simulink model "CC_Flight_Simulation"  (R2020a)
settings: Solver=VariableStepAuto  StartTime=0.0  StopTime=55  RelTol=1e-3
values from neighbouring files (symbols this model uses):
  Ar = 0.0126676869774    [barrowaman.mat]
  CD_data = [0.48 0.48 0.47 0.46 0.45 0.44 0.43 0.42 0.42 0.41 0.4 0.4 ... (150 elements, 150x1)]    [barrowaman.mat]
  CD_input = [0.01 0.02 0.03 0.04 0.05 0.06 0.07 0.08 0.09 0.1 0.11 0.12 ... (150 elements, 150x1)]    [barrowaman.mat]
  CnalfaBody = 2.2 * lTubo    [Barrowman_Equations.m]    (also in barrowaman.mat = -4.333362)
  CnAlfaNose = 2 * pi * (r0^2) / Ar    [Barrowman_Equations.m]    (also in barrowaman.mat = 2)
  Cnalfat = Cnalfat * (1 + r0/(span + r0))    [Barrowman_Equations.m]    (also in barrowaman.mat = 7.14285935703)
  CnAlfaTail = 0    [Barrowman_Equations.m]    (also in barrowaman.mat = -1.06144212288)
  Cndomega = (N * (c1 + c2 + c3))/(Ar * (Lr))    [Barrowman_Equations.m]
  Cnfdelta = N * Y / span    [Barrowman_Equations.m]    (also in barrowaman.mat = 4.20666666667)
  delta = 0.00872664625997    [barrowaman.mat]
  F_data = [3391.768 3665.504 3532.913 3357.551 3199.297 3139.417 2412.304 2130.013 2031.639 346.448 81.266 0 ... (14 elements, 14x1)]    [barrowaman.mat]
  F_input = [0.02 0.057 0.148 0.496 0.817 0.936 1.173 1.501 1.717 1.78 1.812 1.832 ... (14 elements, 14x1)]    [barrowaman.mat]
  Lr = 0.127    [barrowaman.mat]
  mdescarregado = 15.576    [barrowaman.mat]
  MDot_data = [-1.96086837808 -2.11912220509 -2.04246793537 -1.9410866497 -1.84959593916 -1.81497776997 -1.39461503025 -1.23141533755 -1.1745427962 -0.200290505674 -0.0469819662232 0 ... (18 elements, 18x1)]    [barrowaman.mat]
  MDot_input = [0.02 0.057 0.148 0.496 0.817 0.936 1.173 1.501 1.717 1.78 1.812 1.832 ... (18 elements, 18x1)]    [barrowaman.mat]
  r = 0    [Barrowman_Equations.m]    (also in barrowaman.mat = 1.45977011494)
  x_cg = -1.278    [barrowaman.mat]
  XB = -(logiva - logiva/2)    [Barrowman_Equations.m]    (also in barrowaman.mat = 0.279145)
  Xtail = 0    [Barrowman_Equations.m]    (also in barrowaman.mat = -2.55613084112)
  XTB = pos_aletas - (sweep / 3) * ( (Cr + 2 * Ct) / (Cr + Ct) ) + (1/6) * (Cr + Ct - Cr * Ct / (Cr + Ct))    [Barrowman_Equations.m]    (also in barrowaman.mat = -2.37866666667)
  Y = rt + (span/3) * yparcial    [Barrowman_Equations.m]    (also in barrowaman.mat = 0.105166666667)
undefined symbols (not defined in the file or in its folder): F, Light, MIL
libraries: sharedutil x8, aerolibasang x3, aerolibwind2 x3, aerolibanim x1, aerolibatmos2 x1, shared6dof x1
settings Model: Creator=bruno  LastModifiedBy=patri
settings OptimizationCC: LifeSpan=inf
settings DebuggingCC: ArithmeticOperatorsInVariantConditions=warning
settings SFSimCC: CustomCodeUndefinedFunction=UseInterfaceOnly
settings CodeAppCC: StateflowObjectComments=on
settings SimscapeCC: SimscapeNormalizeSystem=off

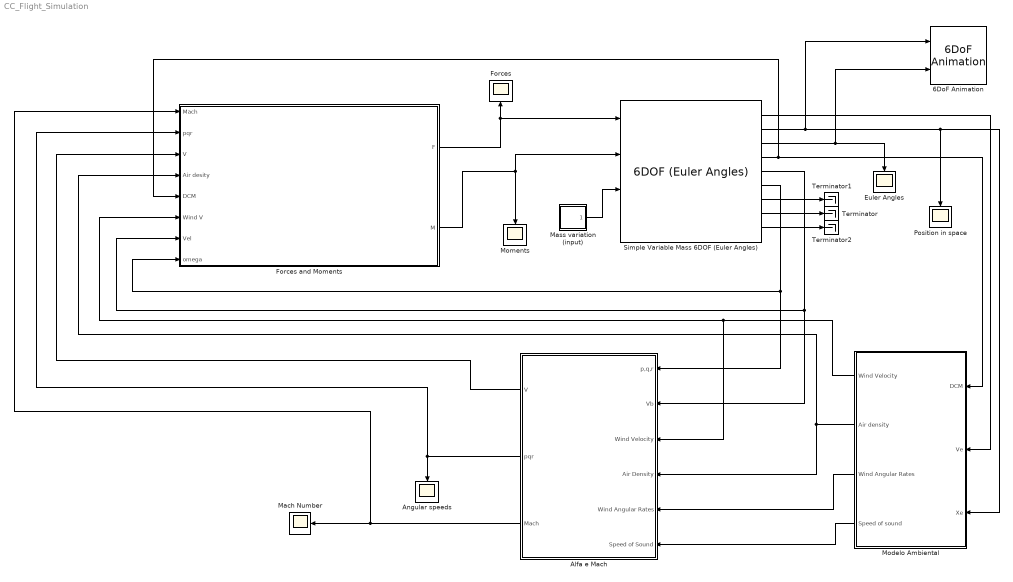
== system CC_Flight_Simulation ==
  6DoF Animation : aerolibanim/6DoF Animation  u1=[0 400 -200 200 0 4000]  u2=0.1  u3=100  u4=[4000 0 -5000]  u5=Fly alongside  u6=[2000 500 -3150]  u7=10  u8=on
  Alfa e Mach : Subsystem
  Angular speeds : Scope
  Euler Angles : Scope
  Forces : Scope
  "Forces and Moments " : Subsystem
  Mach Number : Scope
  Mass variation (input) : Subsystem
  Modelo Ambiental : Subsystem
  Moments : Scope
  "Position in space " : Scope
  Simple Variable Mass 6DOF (Euler Angles) : shared6dof/6DOF (Euler Angles)  units=Metric (MKS)  mtype=Simple Variable  rep=Quaternion  xme_0=[5 0 0]  Vm_0=[20 0 0]  eul_0=[0 -pi/2+pi/30 0]  pm_0=[0 0 0]  mass_0=mcarregado  mass_e=mdescarregado  mass_f=mcarregado  inertia=eye(3)  inertia_e=MatrizDeInerciaDescarregado  inertia_f=MatrizDeInercia  k_quat=1.0  vre_flag=on  abi_flag=off  aMode=aMode  xme_statename=''  Vm_statename=''  eul_statename=''  quat_statename=''  pm_statename=''  mass_statename=''
      settings: SourceProductBaseCode=AE,PW,MT,VE,VP
  Terminator : Terminator
  Terminator1 : Terminator
  Terminator2 : Terminator
  wires:
  Simple Variable Mass 6DOF (Euler Angles)/4 -> Modelo Ambiental/1(DCM), "Forces and Moments "/5(DCM)
  Simple Variable Mass 6DOF (Euler Angles)/1 -> Modelo Ambiental/2(Ve)
  Simple Variable Mass 6DOF (Euler Angles)/2 -> 6DoF Animation/1, "Position in space "/1, Modelo Ambiental/3(Xe)
  Modelo Ambiental/2(Air density) -> Alfa e Mach/4(Air Density), "Forces and Moments "/4(Air desity)
  Modelo Ambiental/1(Wind Velocity) -> Alfa e Mach/3(Wind Velocity), "Forces and Moments "/6("Wind V ")
  Simple Variable Mass 6DOF (Euler Angles)/5 -> "Forces and Moments "/7("Vel "), Alfa e Mach/2(Vb)
  Simple Variable Mass 6DOF (Euler Angles)/6 -> "Forces and Moments "/8(omega), Alfa e Mach/1(p,q,r)
  Modelo Ambiental/4(Speed of sound) -> Alfa e Mach/6(Speed of Sound)
  Modelo Ambiental/3(Wind Angular Rates) -> Alfa e Mach/5(Wind Angular Rates)
  Alfa e Mach/3(Mach) -> "Forces and Moments "/1(Mach), Mach Number/1
  Alfa e Mach/2(pqr) -> "Forces and Moments "/2(pqr), Angular speeds/1
  Alfa e Mach/1(V) -> "Forces and Moments "/3("V ")
  Simple Variable Mass 6DOF (Euler Angles)/3 -> 6DoF Animation/2, Euler Angles/1
  "Forces and Moments "/1(F) -> Simple Variable Mass 6DOF (Euler Angles)/1, Forces/1
  Simple Variable Mass 6DOF (Euler Angles)/7 -> Terminator1/1
  Simple Variable Mass 6DOF (Euler Angles)/8 -> Terminator/1
  Simple Variable Mass 6DOF (Euler Angles)/9 -> Terminator2/1
  "Forces and Moments "/2(M) -> Simple Variable Mass 6DOF (Euler Angles)/2, Moments/1
  Mass variation (input)/1("dM/dt ") -> Simple Variable Mass 6DOF (Euler Angles)/3

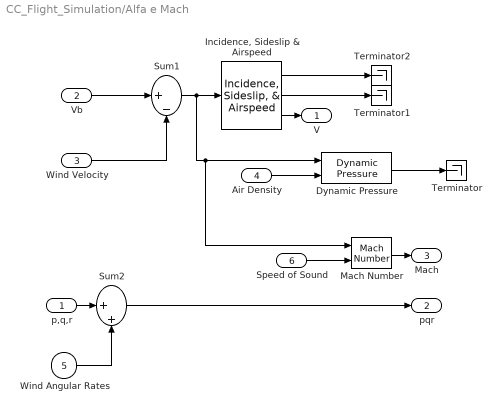
== system CC_Flight_Simulation/Alfa e Mach ==
  p,q,r : Inport
  Vb : Inport  Port=2
  Wind Velocity : Inport  Port=3
  Air Density : Inport  Port=4
  Wind Angular Rates : Inport  Port=5
  Speed of Sound : Inport  Port=6  Unit=m/s
  Dynamic Pressure : aerolibasang/Dynamic Pressure
  "Incidence, Sideslip & Airspeed" : aerolibasang/Incidence, Sideslip, & Airspeed
  Mach Number : aerolibasang/Mach Number
      settings: SourceProductBaseCode=AE
  Sum1 : Sum  Inputs=|+-  InputSameDT=on  SaturateOnIntegerOverflow=on  OutDataTypeStr=Inherit: Same as first input
  Sum2 : Sum  Inputs=|++  InputSameDT=on  SaturateOnIntegerOverflow=on  OutDataTypeStr=Inherit: Same as first input
  Terminator : Terminator
  Terminator1 : Terminator
  Terminator2 : Terminator
  V : Outport  VectorParamsAs1DForOutWhenUnconnected=off
  pqr : Outport  Port=2  VectorParamsAs1DForOutWhenUnconnected=off
  Mach : Outport  Port=3  VectorParamsAs1DForOutWhenUnconnected=off
  wires:
  Wind Velocity/1 -> Sum1/2
  Air Density/1 -> Dynamic Pressure/2
  Dynamic Pressure/1 -> Terminator/1
  "Incidence, Sideslip & Airspeed"/3 -> V/1
  p,q,r/1 -> Sum2/1
  Wind Angular Rates/1 -> Sum2/2
  Sum2/1 -> pqr/1
  Vb/1 -> Sum1/1
  Mach Number/1 -> Mach/1
  Sum1/1 -> Mach Number/1, Dynamic Pressure/1, "Incidence, Sideslip & Airspeed"/1
  Speed of Sound/1 -> Mach Number/2
  "Incidence, Sideslip & Airspeed"/2 -> Terminator1/1
  "Incidence, Sideslip & Airspeed"/1 -> Terminator2/1

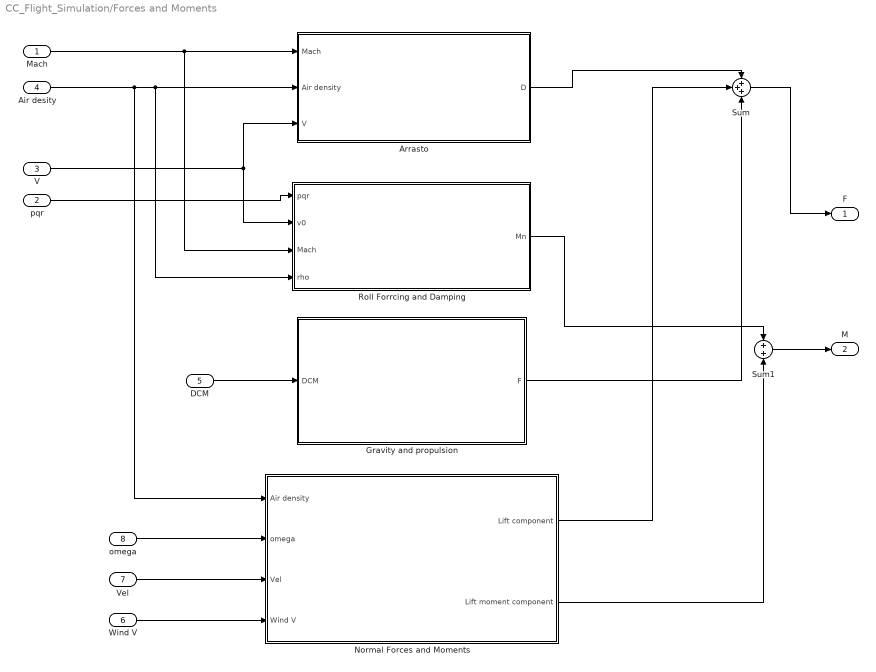
== system CC_Flight_Simulation/Forces and Moments  ==
  Mach : Inport
  pqr : Inport  Port=2
  "V " : Inport  Port=3
  Air desity : Inport  Port=4
  DCM : Inport  Port=5
  "Wind V " : Inport  Port=6
  "Vel " : Inport  Port=7
  omega : Inport  Port=8
  Arrasto : Subsystem
  Gravity and propulsion : Subsystem
  Normal Forces and Moments : Subsystem
  Roll Forrcing and Damping : Subsystem
  Sum : Sum  Inputs=3
  Sum1 : Sum  Inputs=2
  F : Outport  VectorParamsAs1DForOutWhenUnconnected=off
  M : Outport  Port=2  VectorParamsAs1DForOutWhenUnconnected=off
  wires:
  Mach/1 -> Roll Forrcing and Damping/3("Mach "), Arrasto/1(Mach)
  pqr/1 -> Roll Forrcing and Damping/1(pqr)
  "V "/1 -> Roll Forrcing and Damping/2("v0 "), Arrasto/3("V ")
  Air desity/1 -> Roll Forrcing and Damping/4(rho), Arrasto/2(Air density), Normal Forces and Moments/1(Air density)
  Sum/1 -> F/1
  Gravity and propulsion/1(F) -> Sum/3
  DCM/1 -> Gravity and propulsion/1(DCM)
  Arrasto/1(D) -> Sum/1
  Roll Forrcing and Damping/1(Mn) -> Sum1/1
  Sum1/1 -> M/1
  omega/1 -> Normal Forces and Moments/2(omega)
  "Vel "/1 -> Normal Forces and Moments/3("Vel ")
  "Wind V "/1 -> Normal Forces and Moments/4("Wind V ")
  Normal Forces and Moments/1("Lift component ") -> Sum/2
  Normal Forces and Moments/2("Lift moment component ") -> Sum1/2

== system CC_Flight_Simulation/Mass variation (input) ==
  1-D Lookup Table1 : Lookup_n-D  NumberOfTableDimensions=1  BreakpointsForDimension1=MDot_input  Table=MDot_data  InternalRulePriority=Speed  RndMeth=Simplest  InputSameDT=on
  Clock : Clock
  Forças1 : Scope
  "dM/dt " : Outport  VectorParamsAs1DForOutWhenUnconnected=off
  wires:
  1-D Lookup Table1/1 -> "dM/dt "/1, Forças1/1
  Clock/1 -> 1-D Lookup Table1/1

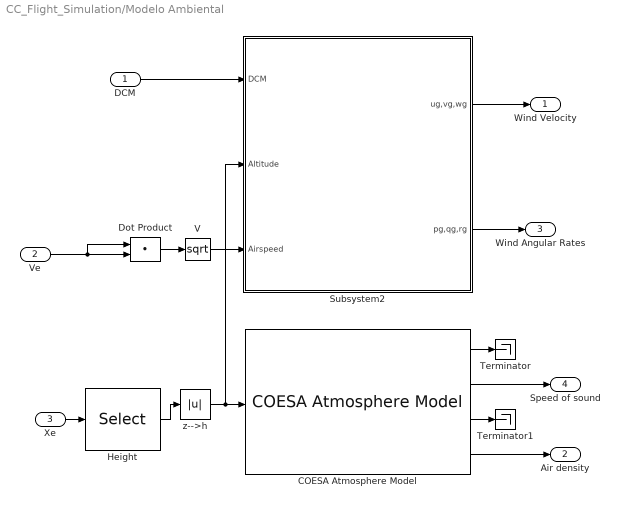
== system CC_Flight_Simulation/Modelo Ambiental ==
  DCM : Inport
  Ve : Inport  Port=2
  Xe : Inport  Port=3
  COESA Atmosphere Model : aerolibatmos2/COESA Atmosphere Model  units=Metric (MKS)  spec=1976 COESA-extended U.S. Standard Atmosphere  model=Profile  profile_var=High temperature  profile_percent=10%  profile_alt=5 km (16404 ft)  envelope_var=High temperature  envelope_percent=1%  action=None
  Dot Product : DotProduct  SaturateOnIntegerOverflow=on  OutDataTypeStr=Inherit: Inherit via internal rule
  Height : Selector  InputPortWidth=3  IndexOptions=Index vector (dialog)  Indices=[3]  OutputSizes=1
  Subsystem2 : Subsystem
  Terminator : Terminator
  Terminator1 : Terminator
  V : Math  Operator=sqrt  SignedPower=on  SaturateOnIntegerOverflow=on
  z-->h : Abs  SaturateOnIntegerOverflow=on
  Wind Velocity : Outport  VectorParamsAs1DForOutWhenUnconnected=off
  Air density : Outport  Port=2  VectorParamsAs1DForOutWhenUnconnected=off
  Wind Angular Rates : Outport  Port=3  VectorParamsAs1DForOutWhenUnconnected=off
  Speed of sound : Outport  Port=4  VectorParamsAs1DForOutWhenUnconnected=off
  wires:
  z-->h/1 -> Subsystem2/2(Altitude), COESA Atmosphere Model/1
  Subsystem2/1(ug,vg,wg) -> Wind Velocity/1
  Subsystem2/2(pg,qg,rg) -> Wind Angular Rates/1
  DCM/1 -> Subsystem2/1(DCM)
  Ve/1 -> Dot Product/1, Dot Product/2
  Dot Product/1 -> V/1
  V/1 -> Subsystem2/3(Airspeed)
  COESA Atmosphere Model/2 -> Speed of sound/1
  COESA Atmosphere Model/3 -> Terminator1/1
  COESA Atmosphere Model/1 -> Terminator/1
  COESA Atmosphere Model/4 -> Air density/1
  Height/1 -> z-->h/1
  Xe/1 -> Height/1

== system CC_Flight_Simulation/Forces and Moments /Arrasto ==
  Mach : Inport
  Air density : Inport  Port=2
  "V " : Inport  Port=3
  1-D Lookup Table1 : Lookup_n-D  NumberOfTableDimensions=1  BreakpointsForDimension1=CD_input  Table=CD_data  InternalRulePriority=Speed  RndMeth=Simplest  InputSameDT=on
  Constant4 : Constant  Value=1/2
  Constant5 : Constant  Value=Ar
  Drag1 : Product  Inputs=6
  Gain : Gain  Gain=[-1 0 0]
  Scope : Scope
  D : Outport  VectorParamsAs1DForOutWhenUnconnected=off
  wires:
  Mach/1 -> 1-D Lookup Table1/1
  Gain/1 -> Scope/1, D/1
  Drag1/1 -> Gain/1
  Constant4/1 -> Drag1/1
  1-D Lookup Table1/1 -> Drag1/2
  "V "/1 -> Drag1/5, Drag1/4
  Constant5/1 -> Drag1/6
  Air density/1 -> Drag1/3

== system CC_Flight_Simulation/Forces and Moments /Gravity and propulsion ==
  DCM : Inport
  "Gravidade " : Subsystem
  "Propulsão " : Subsystem
  Scope : Scope
  Scope1 : Scope
  Sum : Sum  Inputs=|++
  F : Outport  VectorParamsAs1DForOutWhenUnconnected=off
  wires:
  Sum/1 -> F/1
  "Propulsão "/1(F motor) -> Scope1/1, Sum/1
  DCM/1 -> "Gravidade "/1(DCM)
  "Gravidade "/1("F_gravidade ") -> Sum/2, Scope/1

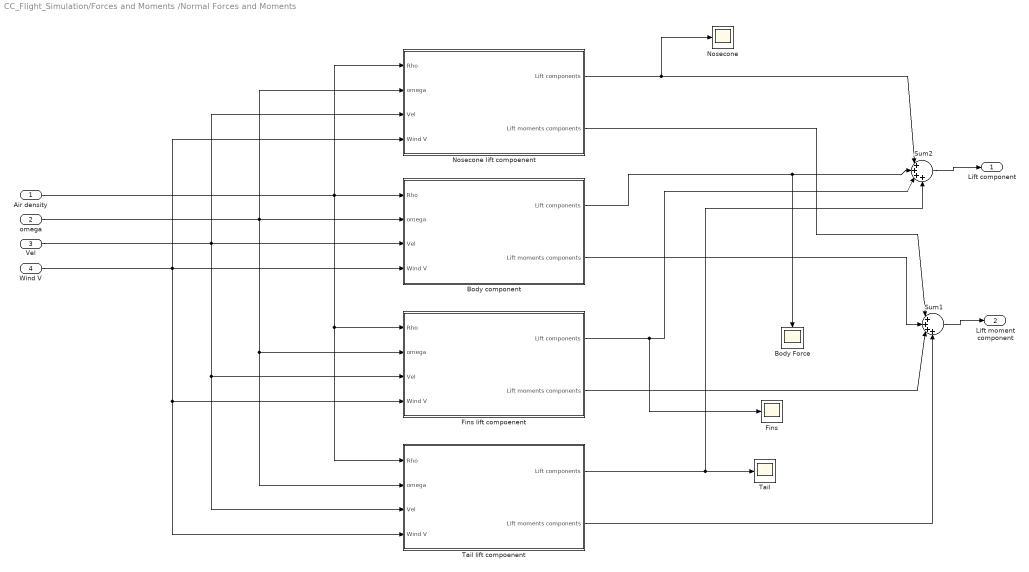
== system CC_Flight_Simulation/Forces and Moments /Normal Forces and Moments ==
  Air density : Inport
  omega : Inport  Port=2
  "Vel " : Inport  Port=3
  "Wind V " : Inport  Port=4
  Body Force : Scope
  Body component : Subsystem
  Fins : Scope
  "Fins lift compoenent " : Subsystem
  Nosecone : Scope
  Nosecone lift compoenent : Subsystem
  Sum1 : Sum  Inputs=|++++
  Sum2 : Sum  Inputs=|++++
  Tail : Scope
  "Tail lift compoenent " : Subsystem
  "Lift component " : Outport  VectorParamsAs1DForOutWhenUnconnected=off
  "Lift moment component " : Outport  Port=2  VectorParamsAs1DForOutWhenUnconnected=off
  wires:
  "Vel "/1 -> "Fins lift compoenent "/3("Vel "), "Tail lift compoenent "/3("Vel "), Body component/3("Vel "), Nosecone lift compoenent/3("Vel ")
  omega/1 -> "Fins lift compoenent "/2(omega), "Tail lift compoenent "/2(omega), Body component/2(omega), Nosecone lift compoenent/2(omega)
  "Wind V "/1 -> "Fins lift compoenent "/4("Wind V "), "Tail lift compoenent "/4("Wind V "), Body component/4("Wind V "), Nosecone lift compoenent/4("Wind V ")
  Air density/1 -> "Fins lift compoenent "/1(Rho), "Tail lift compoenent "/1(Rho), Body component/1(Rho), Nosecone lift compoenent/1(Rho)
  Nosecone lift compoenent/1("Lift components ") -> Nosecone/1, Sum2/1
  Sum1/1 -> "Lift moment component "/1
  Sum2/1 -> "Lift component "/1
  Nosecone lift compoenent/2("Lift moments components ") -> Sum1/1
  Body component/1("Lift components ") -> Sum2/2, Body Force/1
  Body component/2("Lift moments components ") -> Sum1/2
  "Fins lift compoenent "/1("Lift components ") -> Fins/1, Sum2/3
  "Fins lift compoenent "/2("Lift moments components ") -> Sum1/3
  "Tail lift compoenent "/1("Lift components ") -> Tail/1, Sum2/4
  "Tail lift compoenent "/2("Lift moments components ") -> Sum1/4

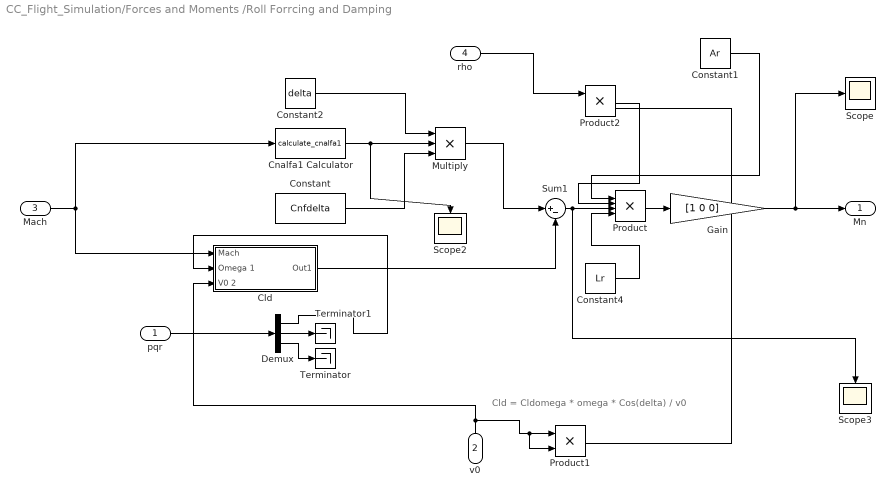
== system CC_Flight_Simulation/Forces and Moments /Roll Forrcing and Damping ==
  note: Cld = Cldomega * omega * Cos(delta) / v0
  pqr : Inport
  "v0 " : Inport  Port=2
  "Mach " : Inport  Port=3
  rho : Inport  Port=4
  "Cld " : Subsystem
  "Cnalfa1 Calculator " : MATLABFcn  MATLABFcn=calculate_cnalfa1
  Constant : Constant  Value=Cnfdelta
  Constant1 : Constant  Value=Ar
  Constant2 : Constant  Value=delta
  Constant4 : Constant  Value=Lr
  Demux : Demux  Outputs=3
  Gain : Gain  Gain=[1 0 0]
  "Multiply " : Product  Inputs=***
  Product : Product  Inputs=4
  Product1 : Product
  Product2 : Product
  Scope : Scope
  Scope2 : Scope
  Scope3 : Scope
  Sum1 : Sum  Inputs=|+-
  Terminator : Terminator
  Terminator1 : Terminator
  Mn : Outport  VectorParamsAs1DForOutWhenUnconnected=off
  wires:
  Constant2/1 -> "Multiply "/1
  "v0 "/1 -> "Cld "/3(V0 2), Product1/2, Product1/1
  "Multiply "/1 -> Sum1/1
  pqr/1 -> Demux/1
  Constant/1 -> "Multiply "/3
  Demux/2 -> Terminator1/1
  Gain/1 -> Scope/1, Mn/1
  Demux/3 -> Terminator/1
  Demux/1 -> "Cld "/2(Omega 1)
  "Mach "/1 -> "Cnalfa1 Calculator "/1, "Cld "/1("Mach ")
  "Cnalfa1 Calculator "/1 -> Scope2/1, "Multiply "/2
  Product/1 -> Gain/1
  Constant1/1 -> Product/1
  Constant4/1 -> Product/4
  Product1/1 -> Product2/2
  rho/1 -> Product2/1
  Product2/1 -> Product/2
  "Cld "/1(Out1) -> Sum1/2
  Sum1/1 -> Scope3/1, Product/3

== system CC_Flight_Simulation/Modelo Ambiental/Subsystem2 ==
  DCM : Inport
  Altitude : Inport  Port=2
  Airspeed : Inport  Port=3
  Discrete Wind Gust Model - On : aerolibwind2/Discrete Wind Gust Model  units=Metric (MKS)  Gx=on  Gy=on  Gz=on  t_0=20  d_m=[120 120 80]  v_m=[3.5 3.0 3.0]
  Dryden Wind Turbulence Model (Continuous (+q -r)) : aerolibwind2/Dryden Wind Turbulence Model  (Continuous (+q -r))  Commented=on  units=Metric (MKS)  spec=MIL-F-8785C  model=Continuous Dryden (+q -r)  W20=5  Wdeg=0  TurbProb=10^-2 - Light  L_high=533.4  Wingspan=4  ts=0.1  Seed=[23341 23342 23343 23344]  T_on=on
  Sum1 : Sum  Inputs=+++  InputSameDT=on  SaturateOnIntegerOverflow=on  OutDataTypeStr=Inherit: Same as first input
  Wind Shear Model : aerolibwind2/Wind Shear Model  units=Metric (MKS)  phase=Category C - Terminal Flight Phase  W_20=1  Wdeg=0
  ug,vg,wg : Outport  VectorParamsAs1DForOutWhenUnconnected=off
  pg,qg,rg : Outport  Port=2  VectorParamsAs1DForOutWhenUnconnected=off
  wires:
  Dryden Wind Turbulence Model (Continuous (+q -r))/2 -> pg,qg,rg/1
  Wind Shear Model/1 -> Sum1/1
  Dryden Wind Turbulence Model (Continuous (+q -r))/1 -> Sum1/2
  Discrete Wind Gust Model - On/1 -> Sum1/3
  DCM/1 -> Dryden Wind Turbulence Model (Continuous (+q -r))/3, Wind Shear Model/2
  Airspeed/1 -> Dryden Wind Turbulence Model (Continuous (+q -r))/2, Discrete Wind Gust Model - On/1
  Sum1/1 -> ug,vg,wg/1
  Altitude/1 -> Dryden Wind Turbulence Model (Continuous (+q -r))/1, Wind Shear Model/1

== system CC_Flight_Simulation/Forces and Moments /Gravity and propulsion/Gravidade  ==
  DCM : Inport
  Constant1 : Constant  Value=9.81*mdescarregado
  Gain3 : Gain  Gain=[0 0 -1]
  Inertial to Body : Product  Multiplication=Matrix(*)  InputSameDT=on  SaturateOnIntegerOverflow=on  OutDataTypeStr=Inherit: Same as first input
  "F_gravidade " : Outport  VectorParamsAs1DForOutWhenUnconnected=off
  wires:
  Inertial to Body/1 -> "F_gravidade "/1
  DCM/1 -> Inertial to Body/1
  Gain3/1 -> Inertial to Body/2
  Constant1/1 -> Gain3/1

== system CC_Flight_Simulation/Forces and Moments /Gravity and propulsion/Propulsão  ==
  1-D Lookup Table : Lookup_n-D  NumberOfTableDimensions=1  BreakpointsForDimension1=F_input  Table=F_data  InternalRulePriority=Speed  RndMeth=Simplest  InputSameDT=on
  Clock1 : Clock
  Gain : Gain  Gain=[1 0 0]
  Scope : Scope
  F motor : Outport  VectorParamsAs1DForOutWhenUnconnected=off
  wires:
  Clock1/1 -> 1-D Lookup Table/1
  1-D Lookup Table/1 -> Gain/1
  Gain/1 -> Scope/1, F motor/1

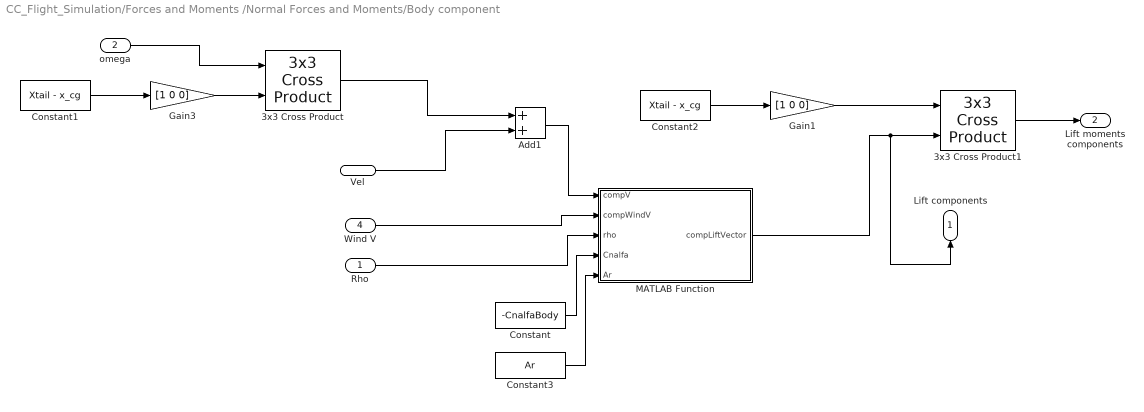
== system CC_Flight_Simulation/Forces and Moments /Normal Forces and Moments/Body component ==
  Rho : Inport
  omega : Inport  Port=2
  "Vel " : Inport  Port=3
  "Wind V " : Inport  Port=4
  3x3 Cross Product : sharedutil/3x3 Cross Product  aMode=aMode
      settings: SourceProductBaseCode=AE,PW,MT,VE,VP
  3x3 Cross Product1 : sharedutil/3x3 Cross Product  aMode=aMode
      settings: SourceProductBaseCode=AE,PW,MT,VE,VP
  Add1 : Sum
  Constant : Constant  Value=-CnalfaBody
  Constant1 : Constant  Value=Xtail - x_cg
  Constant2 : Constant  Value=Xtail - x_cg
  Constant3 : Constant  Value=Ar
  Gain1 : Gain  Gain=[1 0 0]
  Gain3 : Gain  Gain=[1 0 0]
  MATLAB Function : MATLAB Function  TreatAsAtomicUnit=on
  "Lift components " : Outport  VectorParamsAs1DForOutWhenUnconnected=off
  "Lift moments components " : Outport  Port=2  VectorParamsAs1DForOutWhenUnconnected=off
  wires:
  omega/1 -> 3x3 Cross Product/1
  "Vel "/1 -> Add1/2
  MATLAB Function/1(compLiftVector) -> 3x3 Cross Product1/2, "Lift components "/1
  3x3 Cross Product/1 -> Add1/1
  Add1/1 -> MATLAB Function/1(compV)
  3x3 Cross Product1/1 -> "Lift moments components "/1
  Constant1/1 -> Gain3/1
  Gain3/1 -> 3x3 Cross Product/2
  Constant2/1 -> Gain1/1
  Gain1/1 -> 3x3 Cross Product1/1
  "Wind V "/1 -> MATLAB Function/2(compWindV)
  Rho/1 -> MATLAB Function/3(rho)
  Constant/1 -> MATLAB Function/4(Cnalfa)
  Constant3/1 -> MATLAB Function/5(Ar)

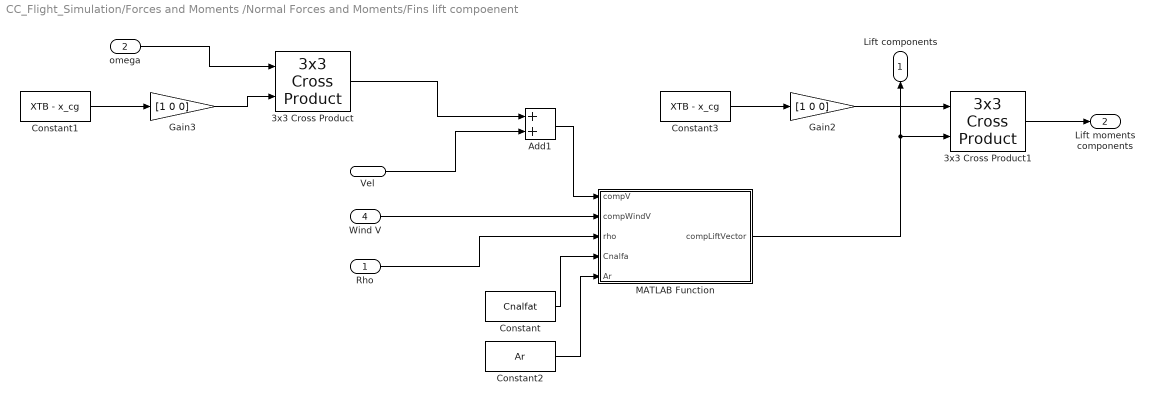
== system CC_Flight_Simulation/Forces and Moments /Normal Forces and Moments/Fins lift compoenent  ==
  Rho : Inport
  omega : Inport  Port=2
  "Vel " : Inport  Port=3
  "Wind V " : Inport  Port=4
  3x3 Cross Product : sharedutil/3x3 Cross Product  aMode=aMode
      settings: SourceProductBaseCode=AE,PW,MT,VE,VP
  3x3 Cross Product1 : sharedutil/3x3 Cross Product  aMode=aMode
      settings: SourceProductBaseCode=AE,PW,MT,VE,VP
  Add1 : Sum
  Constant : Constant  Value=Cnalfat
  Constant1 : Constant  Value=XTB - x_cg
  Constant2 : Constant  Value=Ar
  Constant3 : Constant  Value=XTB - x_cg
  Gain2 : Gain  Gain=[1 0 0]
  Gain3 : Gain  Gain=[1 0 0]
  MATLAB Function : MATLAB Function  TreatAsAtomicUnit=on
  "Lift components " : Outport  VectorParamsAs1DForOutWhenUnconnected=off
  "Lift moments components " : Outport  Port=2  VectorParamsAs1DForOutWhenUnconnected=off
  wires:
  omega/1 -> 3x3 Cross Product/1
  "Vel "/1 -> Add1/2
  MATLAB Function/1(compLiftVector) -> 3x3 Cross Product1/2, "Lift components "/1
  Gain3/1 -> 3x3 Cross Product/2
  "Wind V "/1 -> MATLAB Function/2(compWindV)
  3x3 Cross Product/1 -> Add1/1
  Add1/1 -> MATLAB Function/1(compV)
  Rho/1 -> MATLAB Function/3(rho)
  3x3 Cross Product1/1 -> "Lift moments components "/1
  Constant1/1 -> Gain3/1
  Constant3/1 -> Gain2/1
  Gain2/1 -> 3x3 Cross Product1/1
  Constant/1 -> MATLAB Function/4(Cnalfa)
  Constant2/1 -> MATLAB Function/5(Ar)

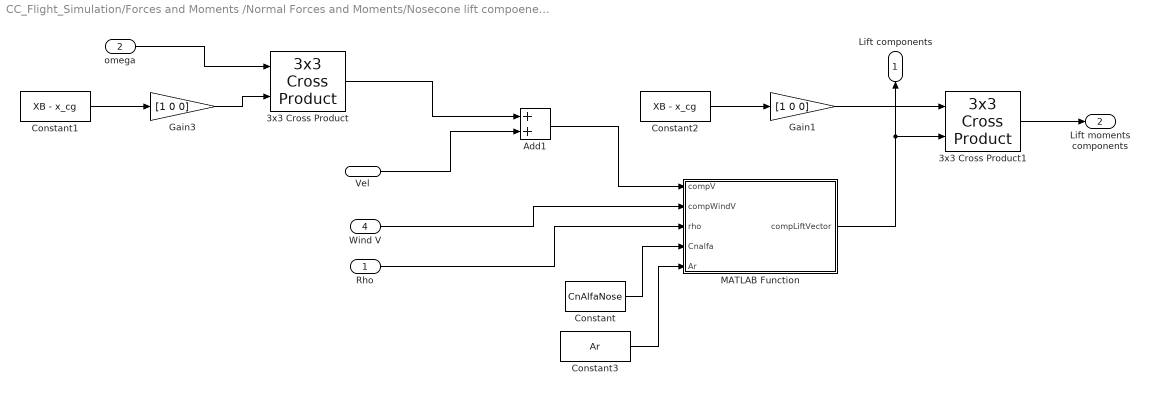
== system CC_Flight_Simulation/Forces and Moments /Normal Forces and Moments/Nosecone lift compoenent ==
  Rho : Inport
  omega : Inport  Port=2
  "Vel " : Inport  Port=3
  "Wind V " : Inport  Port=4
  3x3 Cross Product : sharedutil/3x3 Cross Product  aMode=aMode
      settings: SourceProductBaseCode=AE,PW,MT,VE,VP
  3x3 Cross Product1 : sharedutil/3x3 Cross Product  aMode=aMode
      settings: SourceProductBaseCode=AE,PW,MT,VE,VP
  Add1 : Sum
  Constant : Constant  Value=CnAlfaNose
  Constant1 : Constant  Value=XB - x_cg
  Constant2 : Constant  Value=XB - x_cg
  Constant3 : Constant  Value=Ar
  Gain1 : Gain  Gain=[1 0 0]
  Gain3 : Gain  Gain=[1 0 0]
  MATLAB Function : MATLAB Function  TreatAsAtomicUnit=on
  "Lift components " : Outport  VectorParamsAs1DForOutWhenUnconnected=off
  "Lift moments components " : Outport  Port=2  VectorParamsAs1DForOutWhenUnconnected=off
  wires:
  omega/1 -> 3x3 Cross Product/1
  "Vel "/1 -> Add1/2
  MATLAB Function/1(compLiftVector) -> 3x3 Cross Product1/2, "Lift components "/1
  Gain3/1 -> 3x3 Cross Product/2
  "Wind V "/1 -> MATLAB Function/2(compWindV)
  Constant1/1 -> Gain3/1
  3x3 Cross Product/1 -> Add1/1
  Add1/1 -> MATLAB Function/1(compV)
  Rho/1 -> MATLAB Function/3(rho)
  3x3 Cross Product1/1 -> "Lift moments components "/1
  Constant2/1 -> Gain1/1
  Gain1/1 -> 3x3 Cross Product1/1
  Constant/1 -> MATLAB Function/4(Cnalfa)
  Constant3/1 -> MATLAB Function/5(Ar)

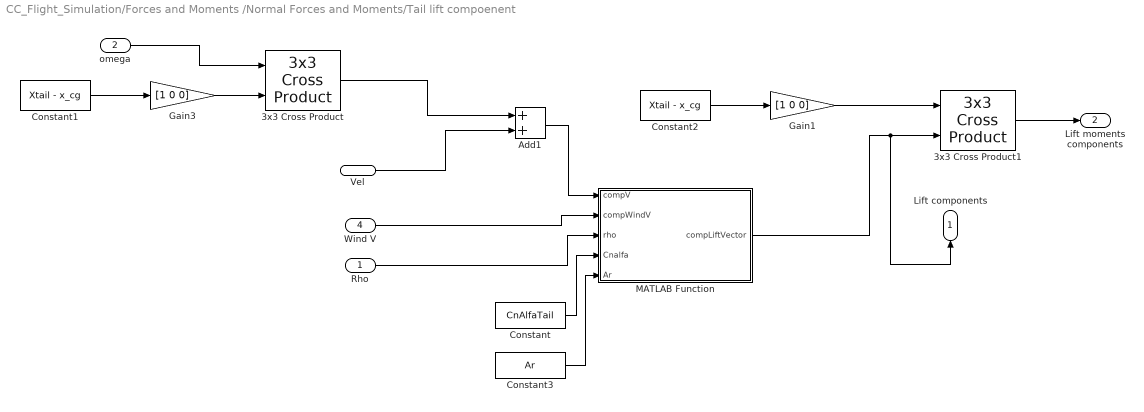
== system CC_Flight_Simulation/Forces and Moments /Normal Forces and Moments/Tail lift compoenent  ==
  Rho : Inport
  omega : Inport  Port=2
  "Vel " : Inport  Port=3
  "Wind V " : Inport  Port=4
  3x3 Cross Product : sharedutil/3x3 Cross Product  aMode=aMode
      settings: SourceProductBaseCode=AE,PW,MT,VE,VP
  3x3 Cross Product1 : sharedutil/3x3 Cross Product  aMode=aMode
      settings: SourceProductBaseCode=AE,PW,MT,VE,VP
  Add1 : Sum
  Constant : Constant  Value=CnAlfaTail
  Constant1 : Constant  Value=Xtail - x_cg
  Constant2 : Constant  Value=Xtail - x_cg
  Constant3 : Constant  Value=Ar
  Gain1 : Gain  Gain=[1 0 0]
  Gain3 : Gain  Gain=[1 0 0]
  MATLAB Function : MATLAB Function  TreatAsAtomicUnit=on
  "Lift components " : Outport  VectorParamsAs1DForOutWhenUnconnected=off
  "Lift moments components " : Outport  Port=2  VectorParamsAs1DForOutWhenUnconnected=off
  wires:
  omega/1 -> 3x3 Cross Product/1
  "Vel "/1 -> Add1/2
  MATLAB Function/1(compLiftVector) -> 3x3 Cross Product1/2, "Lift components "/1
  3x3 Cross Product/1 -> Add1/1
  Add1/1 -> MATLAB Function/1(compV)
  3x3 Cross Product1/1 -> "Lift moments components "/1
  Constant1/1 -> Gain3/1
  Gain3/1 -> 3x3 Cross Product/2
  Constant2/1 -> Gain1/1
  Gain1/1 -> 3x3 Cross Product1/1
  "Wind V "/1 -> MATLAB Function/2(compWindV)
  Rho/1 -> MATLAB Function/3(rho)
  Constant/1 -> MATLAB Function/4(Cnalfa)
  Constant3/1 -> MATLAB Function/5(Ar)

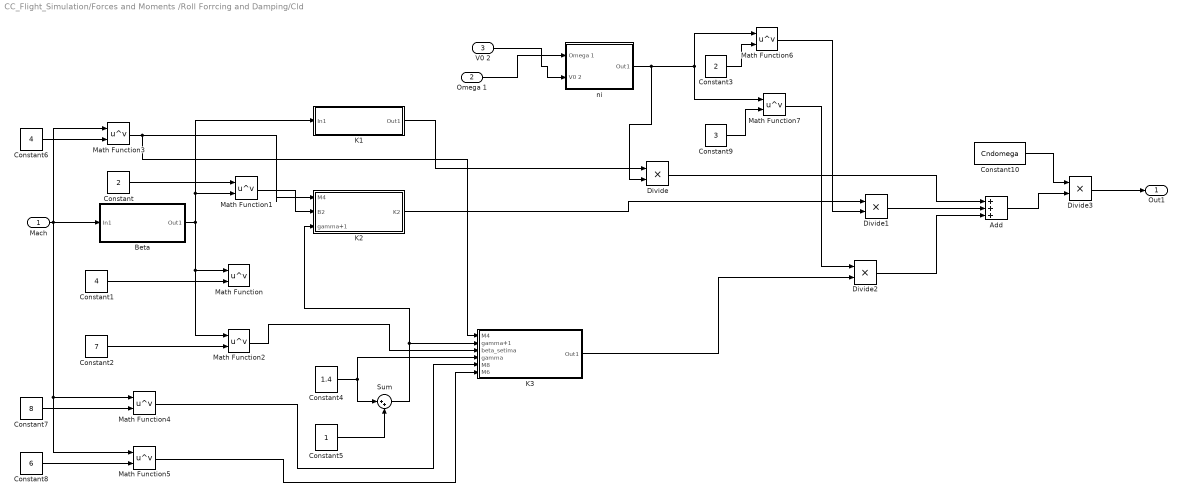
== system CC_Flight_Simulation/Forces and Moments /Roll Forrcing and Damping/Cld  ==
  "Mach " : Inport
  Omega 1 : Inport  Port=2
  V0 2 : Inport  Port=3
  Add : Sum  Inputs=+++
  Beta : Subsystem
  Constant : Constant  Value=2
  Constant1 : Constant  Value=4
  Constant10 : Constant  Value=Cndomega
  Constant2 : Constant  Value=7
  Constant3 : Constant  Value=2
  Constant4 : Constant  Value=1.4
  Constant5 : Constant
  Constant6 : Constant  Value=4
  Constant7 : Constant  Value=8
  Constant8 : Constant  Value=6
  Constant9 : Constant  Value=3
  Divide{,1..3} (4 alike) : Product  Inputs=**
  K1 : Subsystem
  K2 : Subsystem
  K3 : Subsystem
  Math Function{,1..7} (8 alike) : Math  Operator=pow  SaturateOnIntegerOverflow=on
  Sum : Sum  Inputs=|++
  ni : Subsystem
  Out1 : Outport  VectorParamsAs1DForOutWhenUnconnected=off
  wires:
  Divide3/1 -> Out1/1
  "Mach "/1 -> Beta/1(In1), Math Function5/1, Math Function4/1, Math Function3/1
  Constant/1 -> Math Function1/1
  Beta/1(Out1) -> K1/1(In1), Math Function1/2, Math Function/1, Math Function2/1
  Constant1/1 -> Math Function/2
  Constant2/1 -> Math Function2/2
  Constant5/1 -> Sum/2
  Constant4/1 -> K3/4(gamma), Sum/1
  Constant6/1 -> Math Function3/2
  Constant7/1 -> Math Function4/2
  Constant8/1 -> Math Function5/2
  Math Function3/1 -> K3/1(M4), K2/1(" M4")
  Math Function1/1 -> K2/2(B2)
  Sum/1 -> K2/3(gamma+1), K3/2(gamma+1)
  Math Function2/1 -> K3/3(beta_setima)
  Math Function4/1 -> K3/5(M8)
  Math Function5/1 -> K3/6(M6)
  K2/1(K2) -> Divide1/1
  K1/1(Out1) -> Divide/1
  K3/1(Out1) -> Divide2/2
  Omega 1/1 -> ni/1(Omega 1)
  V0 2/1 -> ni/2(V0 2)
  ni/1(Out1) -> Divide/2, Math Function7/1, Math Function6/1
  Constant3/1 -> Math Function6/2
  Constant9/1 -> Math Function7/2
  Math Function6/1 -> Divide1/2
  Math Function7/1 -> Divide2/1
  Divide/1 -> Add/1
  Divide1/1 -> Add/2
  Divide2/1 -> Add/3
  Constant10/1 -> Divide3/1
  Add/1 -> Divide3/2

== system CC_Flight_Simulation/Forces and Moments /Roll Forrcing and Damping/Cld /Beta ==
  In1 : Inport
  Abs : Abs
  Constant : Constant
  Constant1 : Constant  Value=2*pi
  Divide : Product  Inputs=*/
  Product : Product
  Sqrt : Sqrt  SaturateOnIntegerOverflow=on
  Subtract : Sum  Inputs=+-
  Out1 : Outport
  wires:
  Product/1 -> Subtract/2
  In1/1 -> Product/1, Product/2
  Subtract/1 -> Abs/1
  Sqrt/1 -> Divide/2
  Constant/1 -> Subtract/1
  Abs/1 -> Sqrt/1
  Constant1/1 -> Divide/1
  Divide/1 -> Out1/1

== system CC_Flight_Simulation/Forces and Moments /Roll Forrcing and Damping/Cld /K1 ==
  In1 : Inport
  Constant3 : Constant  Value=2
  Divide : Product  Inputs=*/
  Out1 : Outport
  wires:
  Constant3/1 -> Divide/1
  Divide/1 -> Out1/1
  In1/1 -> Divide/2

== system CC_Flight_Simulation/Forces and Moments /Roll Forrcing and Damping/Cld /K2 ==
  " M4" : Inport
  B2 : Inport  Port=2
  gamma+1 : Inport  Port=3
  Constant3 : Constant  Value=4
  Divide : Product  Inputs=/*
  Product : Product
  Product1 : Product
  Subtract : Sum  Inputs=-+
  K2 : Outport
  wires:
  Divide/1 -> K2/1
  Constant3/1 -> Product/2
  " M4"/1 -> Product1/1
  gamma+1/1 -> Product1/2
  B2/1 -> Product/1
  Product1/1 -> Subtract/2
  Product/1 -> Divide/1, Subtract/1
  Subtract/1 -> Divide/2

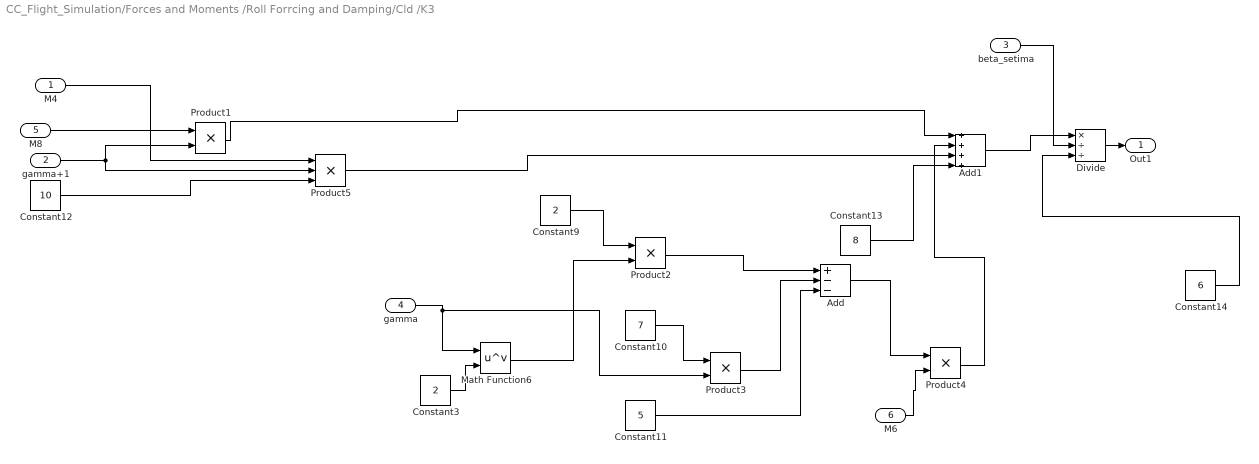
== system CC_Flight_Simulation/Forces and Moments /Roll Forrcing and Damping/Cld /K3 ==
  M4 : Inport
  gamma+1 : Inport  Port=2
  beta_setima : Inport  Port=3
  gamma : Inport  Port=4
  M8 : Inport  Port=5
  M6 : Inport  Port=6
  Add : Sum  Inputs=+--
  Add1 : Sum  Inputs=++++
  Constant10 : Constant  Value=7
  Constant11 : Constant  Value=5
  Constant12 : Constant  Value=10
  Constant13 : Constant  Value=8
  Constant14 : Constant  Value=6
  Constant3 : Constant  Value=2
  Constant9 : Constant  Value=2
  Divide : Product  Inputs=*//
  Math Function6 : Math  Operator=pow  SaturateOnIntegerOverflow=on
  Product{1..4} (4 alike) : Product
  Product5 : Product  Inputs=3
  Out1 : Outport
  wires:
  Product2/1 -> Add/1
  beta_setima/1 -> Divide/2
  Product4/1 -> Add1/2
  Add/1 -> Product4/1
  Constant3/1 -> Math Function6/2
  Divide/1 -> Out1/1
  gamma+1/1 -> Product5/2, Product1/2
  gamma/1 -> Product3/2, Math Function6/1
  Product1/1 -> Add1/1
  Math Function6/1 -> Product2/2
  Constant12/1 -> Product5/3
  Constant11/1 -> Add/3
  Constant10/1 -> Product3/1
  Constant14/1 -> Divide/3
  Constant13/1 -> Add1/4
  Product3/1 -> Add/2
  Constant9/1 -> Product2/1
  Product5/1 -> Add1/3
  Add1/1 -> Divide/1
  M6/1 -> Product4/2
  M4/1 -> Product5/1
  M8/1 -> Product1/1

== system CC_Flight_Simulation/Forces and Moments /Roll Forrcing and Damping/Cld /ni ==
  Omega 1 : Inport
  V0 2 : Inport  Port=2
  Constant3 : Constant  Value=Y
  Divide : Product  Inputs=**/
  Out1 : Outport
  wires:
  Divide/1 -> Out1/1
  Omega 1/1 -> Divide/2
  Constant3/1 -> Divide/1
  V0 2/1 -> Divide/3

== matlab function CC_Flight_Simulation/Forces and Moments /Normal Forces and Moments/Tail lift compoenent /MATLAB Function ==
  data: compV input; compLiftVector output; compWindV input; rho input; Cnalfa input; Ar input
function compLiftVector   = calculate_attack_angle(compV, compWindV, rho, Cnalfa, Ar)
%% Wind Calcs

% Wind relative velocity
compStreamV = compWindV - compV;
% Wind relative velocity magnitude
compStreamSpeed = sqrt(compStreamV(1)^2 + compStreamV(2)^2 + compStreamV(3)^2);
compStreamMagnitudeYZ = (compStreamV(3) ^ 2 + compStreamV(2) ^ 2);
% Normalized vector
compStreamVxBn = compStreamV(1) / compStreamSpeed;

if compStreamMagnitudeYZ ~= 0 && -1 * compStreamVxBn < 1
    %% Angle of attack and component separation
    attack_angle = acos(-compStreamVxBn);
    liftDirNorm =  compStreamMagnitudeYZ^ 0.5;
    y_versor = (compStreamV(2) / liftDirNorm);
    z_versor = (compStreamV(3) / liftDirNorm);

    %% Calculating componentes

    compLift = (0.5 * rho * (compStreamSpeed ^ 2) * Ar * Cnalfa * attack_angle);
    compLiftZB = compLift * z_versor;
    compLiftYB = compLift * y_versor;
else
    compLiftZB = 0;
    compLiftYB = 0;
end
compLiftVector = [0, compLiftYB, compLiftZB];

== matlab function CC_Flight_Simulation/Forces and Moments /Normal Forces and Moments/Nosecone lift compoenent/MATLAB Function ==
  data: compV input; compLiftVector output; compWindV input; rho input; Cnalfa input; Ar input
function compLiftVector   = calculate_attack_angle(compV, compWindV, rho, Cnalfa, Ar)
%% Wind Calcs

% Wind relative velocity
compStreamV = compWindV - compV;
% Wind relative velocity magnitude
compStreamSpeed = sqrt(compStreamV(1)^2 + compStreamV(2)^2 + compStreamV(3)^2);
compStreamMagnitudeYZ = (compStreamV(3) ^ 2 + compStreamV(2) ^ 2);
% Normalized vector
compStreamVxBn = compStreamV(1) / compStreamSpeed;

if compStreamMagnitudeYZ ~= 0 && -1 * compStreamVxBn < 1
    %% Angle of attack and component separation
    attack_angle = acos(-compStreamVxBn);
    liftDirNorm =  compStreamMagnitudeYZ^ 0.5;
    y_versor = (compStreamV(2) / liftDirNorm);
    z_versor = (compStreamV(3) / liftDirNorm);

    %% Calculating componentes

    compLift = (0.5 * rho * (compStreamSpeed ^ 2) * Ar * Cnalfa * attack_angle);
    compLiftZB = compLift * z_versor;
    compLiftYB = compLift * y_versor;
else
    compLiftZB = 0;
    compLiftYB = 0;
end
compLiftVector = [0, compLiftYB, compLiftZB];

== matlab function CC_Flight_Simulation/Forces and Moments /Normal Forces and Moments/Fins lift compoenent /MATLAB Function ==
  data: compV input; compLiftVector output; compWindV input; rho input; Cnalfa input; Ar input
function compLiftVector   = calculate_attack_angle(compV, compWindV, rho, Cnalfa, Ar)
%% Wind Calcs

% Wind relative velocity
compStreamV = compWindV - compV;
% Wind relative velocity magnitude
compStreamSpeed = sqrt(compStreamV(1)^2 + compStreamV(2)^2 + compStreamV(3)^2);
compStreamMagnitudeYZ = (compStreamV(3) ^ 2 + compStreamV(2) ^ 2);
% Normalized vector
compStreamVxBn = compStreamV(1) / compStreamSpeed;

if compStreamMagnitudeYZ ~= 0 && -1 * compStreamVxBn < 1
    %% Angle of attack and component separation
    attack_angle = acos(-compStreamVxBn);
    liftDirNorm =  compStreamMagnitudeYZ^ 0.5;
    y_versor = (compStreamV(2) / liftDirNorm);
    z_versor = (compStreamV(3) / liftDirNorm);

    %% Calculating componentes

    compLift = (0.5 * rho * (compStreamSpeed ^ 2) * Ar * Cnalfa * attack_angle);
    compLiftZB = compLift * z_versor;
    compLiftYB = compLift * y_versor;
else
    compLiftZB = 0;
    compLiftYB = 0;
end
compLiftVector = [0, compLiftYB, compLiftZB];

== matlab function CC_Flight_Simulation/Forces and Moments /Normal Forces and Moments/Body component/MATLAB Function ==
  data: compV input; compLiftVector output; compWindV input; rho input; Cnalfa input; Ar input
function compLiftVector   = calculate_attack_angle(compV, compWindV, rho, Cnalfa, Ar)
%% Wind Calcs

% Wind relative velocity
compStreamV = compWindV - compV;
% Wind relative velocity magnitude
compStreamSpeed = sqrt(compStreamV(1)^2 + compStreamV(2)^2 + compStreamV(3)^2);
compStreamMagnitudeYZ = (compStreamV(3) ^ 2 + compStreamV(2) ^ 2);
% Normalized vector
compStreamVxBn = compStreamV(1) / compStreamSpeed;

if compStreamMagnitudeYZ ~= 0 && -1 * compStreamVxBn < 1
    %% Angle of attack and component separation
    attack_angle = acos(-compStreamVxBn);
    liftDirNorm =  compStreamMagnitudeYZ^ 0.5;
    y_versor = (compStreamV(2) / liftDirNorm);
    z_versor = (compStreamV(3) / liftDirNorm);

    %% Calculating componentes

    compLift = (0.5 * rho * (compStreamSpeed ^ 2) * Ar * Cnalfa * sin(attack_angle) * cos(attack_angle) * attack_angle);
    compLiftZB = compLift * z_versor;
    compLiftYB = compLift * y_versor;
else
    compLiftZB = 0;
    compLiftYB = 0;
end
compLiftVector = [0, compLiftYB, compLiftZB];
